simulink model "T2F_IEEE34bus_v2019b_Phasor_PI_ZIPload"  (R2024a)
settings: Solver=ode4  StartTime=0.0  StopTime=60  FixedStep=Ts  MaxStep=1e-4  RelTol=1e-4
InitFcn:
  | a=1; % Loading Factor
  | Ts=0.1;% For Delay Blocks in Voltage Regulator Controls
  | % phase to sequence conversion of RXB matrices
  | c=1*exp(sqrt(-1)*(120*pi/180));
  | T=[1 1 1;1 c*c c;1 c c*c];
  | Tinv=1/3*[1 1 1;1 c c*c;1 c*c c];
  | 
  | % Simulation data for the IEEE 34 Node Test Feeder model
  | mi2km = 1.60934;%  miles to km conversion
  | ft2km = 0.0003048; % feet to km conversion
  | ms2F = 1*1e-6/(2*pi*60);% microsiemens to Farads conversion
  | 
  | %% Configuration 300 - series reactance - ohm/mile
  | R_300 = [1.3368 0.2101 0.2130;0.2101 1.3238 0.2066;0.2130 0.2066 1.3294];
  | X_300 = [1.3343 0.5779 0.5015;0.5779 1.3569 0.4591;0.5015 0.4591 1.3471];
  | % charging susceptance - microsiemens/mile
  | B_300 = [5.3350 -1.5313 -0.9943;-1.5313 5.0979 -0.6212;-0.9943 -0.6212 4.8880];
  | 
  | R_300 = R_300/mi2km;
  | Rseq=Tinv*R_300*T;
  | R1_300=Rseq(2,2);R0_300=Rseq(1,1);
  | 
  | L_300 = (X_300/(2*pi*60))/mi2km;
  | Lseq=Tinv*L_300*T;
  | L1_300=Lseq(2,2);L0_300=Lseq(1,1);
  | 
  | C_300 =(B_300*ms2F)/mi2km;
  | Cseq=Tinv*C_300*T;
  | C1_300=Cseq(2,2);C0_300=Cseq(1,1);
  | 
  | %% Configuration 301 - series reactance - ohm/mile
  | R_301 = [1.9300 0.2327 0.2359;0.2327 1.9157 0.2288;0.2359 0.2288 1.9219];
  | X_301 = [1.4115 0.6442 0.5691;0.6442 1.4281 0.5238;0.5691 0.5238 1.4209];
  | % charging susceptance - microsiemens/mile
  | B_301 = [5.1207 -1.4364 -0.9402;-1.4364 4.9055 -0.5951;-0.9402 -0.5951 4.7154];
  | 
  | R_301 = R_301/mi2km;
  | Rseq=Tinv*R_301*T;
  | R1_301=Rseq(2,2);R0_301=Rseq(1,1);
  | 
  | L_301 = (X_301/(2*pi*60))/mi2km;
  | Lseq=Tinv*L_301*T;
  | L1_301=Lseq(2,2);L0_301=Lseq(1,1);
  | 
  | C_301 =(B_301*ms2F)/mi2km;
  | Cseq=Tinv*C_301*T;
  | C1_301=Cseq(2,2);C0_301=Cseq(1,1);
  | 
  | %% Configuration 302 - series reactance - ohm/mile
  | R_302 = [2.7995 0 0;0 0 0;0 0 0];
  | X_302 = [1.4855 0 0;0 0 0;0 0 0];
  | % charging susceptance - microsiemens/mile
  | B_302 = [4.2251 0 0;0 0 0;0 0 0];
  | 
  | R_302 = R_302/mi2km;
  | Rseq=Tinv*R_302*T;
  | R1_302=Rseq(2,2);R0_302=Rseq(1,1);
  | 
  | L_302 = (X_302/(2*pi*60))/mi2km;
  | Lseq=Tinv*L_302*T;
  | ... (+41 lines)
values from neighbouring files (symbols this model uses):
  ccc1 = Ccc*d    [CarregaDados1km.m]
  ccc2 = Ccc*d    [CarregaDados1km.m]
  ccc3 = Ccc*d    [CarregaDados1km.m]
  cct1 = Cct*d    [CarregaDados1km.m]
  cct2 = Cct*d    [CarregaDados1km.m]
  cct3 = Cct*d    [CarregaDados1km.m]
  cequa1 = 0    [CarregaDados1km.m]
  cequa2 = 0    [CarregaDados1km.m]
  cequa3 = 0    [CarregaDados1km.m]
  le1 = 1e-10    [CarregaDados1km.m]
  lm1 = (imag(Zm)/(2*pi*f))*d    [CarregaDados1km.m]
  lm2 = (imag(Zm)/(2*pi*f))*d    [CarregaDados1km.m]
  lm3 = (imag(Zm)/(2*pi*f))*d    [CarregaDados1km.m]
  lp1 = (imag(Zp)/(2*pi*f))*d    [CarregaDados1km.m]
  lp2 = (imag(Zp)/(2*pi*f))*d    [CarregaDados1km.m]
  lp3 = (imag(Zp)/(2*pi*f))*d    [CarregaDados1km.m]
  NRE1 = 1e-12    [CarregaDados1km.m]
  rm1 = real(Zm)*d    [CarregaDados1km.m]
  rm2 = real(Zm)*d    [CarregaDados1km.m]
  rm3 = real(Zm)*d    [CarregaDados1km.m]
  rp1 = real(Zp)*d    [CarregaDados1km.m]
  rp2 = real(Zp)*d    [CarregaDados1km.m]
  rp3 = real(Zp)*d    [CarregaDados1km.m]
  rtc0 = 10    [CarregaDados1km.m]
  rtc1 = 10    [CarregaDados1km.m]
  rtc2 = 10    [CarregaDados1km.m]
  rtc3 = 10    [CarregaDados1km.m]
undefined symbols (not defined in the file or in its folder): D11, Delta, find_system, j, le, m1, m2, m3
libraries: spsSeriesRLCBranchLib x192, spsVoltageMeasurementLib x96, spsControlledCurrentSourceLib x90, spsGroundLib x87, spsPowerPhasorLib x57, spsThreePhaseVIMeasurementLib x37, spsThreePhasePISectionLineLib x20, spsCurrentMeasurementLib x12, spsOnDelayLib x12, spsMutualInductanceLib x10, spsThreePhaseSeriesRLCLoadLib x6, spsControlledVoltageSourceLib x6
(part 5 of 8)

== system T2F_IEEE34bus_v2019b_Phasor_PI_ZIPload/Regulator 1 ==
  Mux : Mux  Inputs=3
  Single Phase SVR_A : Subsystem  LoadFcn=find_system(gcs,'FollowLinks', 'on', 'LookUnderMasks', 'all');  mask(Single-Phase OLTC){pNom=5e6/3, fNom=60, vNom=24.9e3/sqrt(3), ctRatio=100, ptRatio=120, DeltaU=0.00625, TapMinMax=[-16 16], InitialTap=12, TapSelectionTime=8, RegulatorOn=on, Regulator=[122/120  2/120  2], Comp=[2.7 1.6]}
      mask prompts: pNom "Nominal Power (VA)"; fNom "Nominal Frequency (Hz)"; vNom "Nominal Voltage (Vrms)"; ctRatio "Primary CT Rating (A)"; ptRatio "PT Ratio"; DeltaU "Voltage Step Per Tap (pu)"; TapMinMax "Minimum and Maximum Tap Positions"; InitialTap "Initial Tap Position"; TapSelectionTime "Tap Selection Time (s)"; RegulatorOn "Voltage Regulator"; Regulator "Voltage Regulator [ Vref(pu) DeadBand(pu)  Delay(s)]"; Comp "Compensator Settings [R (V) X(V)]"
      mask help:
      | Models a single-phase On Load Tap Changer (OLTC). The single-phase secondary of multi-tap winding is modeled with a Variable-Ratio Transformer block.
      |
      | The transformer voltage ratio U2/U1 (in pu) is given by:
      |                 U2/U1= 1+TapPosition*DeltaU
      | Tap position 0 corresponds to nominal voltage ratio.
      |
      | When Voltage regulator is 'on',  voltage regulator asks for a tap change if:
      |                  abs(Vm-Vref)>DeadBand/2  during a time  t > Delay.
      |
      | where 'Vm' is voltage measured at regulating point and Vref is reference voltage.
      | With line drop compensation, Vm=Vsec-Isec(R+jX)
      mask init:
      | RegulatorVref=Regulator(1);
      | RegulatorDeadBand=Regulator(2);
      | RegulatorDelay=Regulator(3);
      | Rc=Comp(1);
      | Xc=Comp(2);
      mask TypeOptions RegulatorOn: off | on
      mask Callback RegulatorOn:
      | tempMaskVis=get_param(gcb,'MaskVisibilities');
      | if strcmp(get_param(gcb,'RegulatorOn'),'on')
      | 	tempMaskVis{11}='on';
      | 	set_param(gcb,'MaskVisibilities',tempMaskVis);
      | else
      | 	tempMaskVis{11}='off';
      | 	set_param(gcb,'MaskVisibilities',tempMaskVis);
      | end
      | if strcmp(get_param(gcb,'RegulatorOn'),'on')
      | 	tempMaskVis{12}='on';
      | 	set_param(gcb,'MaskVisibilities',tempMaskVis);
      | else
      | 	tempMaskVis{12}='off';
      | 	set_param(gcb,'MaskVisibilities',tempMaskVis);
      | end
      mask DialogControl Container8 Prompt: Setup
      mask DialogControl Container13 Prompt: Regulator Parameters
      mask Display:
      | color('blue');
      | r=50;x=40;y=80;
      | th = 0:pi/100:2*pi;
      | f = r * exp(j*th) + x+j*y;
      | plot(real(f), imag(f));
      | color('red');
      | plot([-10 90],[30,130])
      | plot([75 90],[125,130])
      | plot([85 90],[115,130])
      | color('black')
      | port_label('Lconn',1,'S');port_label('Rconn',1,'L');
  Single Phase SVR_B : Subsystem  LoadFcn=find_system(gcs,'FollowLinks', 'on', 'LookUnderMasks', 'all');  mask(Single-Phase OLTC){pNom=5e6/3, fNom=60, vNom=24.9e3/sqrt(3), ctRatio=100, ptRatio=120, DeltaU=0.00625, TapMinMax=[-16 16], InitialTap=5, TapSelectionTime=8, RegulatorOn=on, Regulator=[122/120  2/120  2], Comp=[2.7 1.6]}
      mask prompts: pNom "Nominal Power (VA)"; fNom "Nominal Frequency (Hz)"; vNom "Nominal Voltage (Vrms)"; ctRatio "Primary CT Rating (A)"; ptRatio "PT Ratio"; DeltaU "Voltage Step Per Tap (pu)"; TapMinMax "Minimum and Maximum Tap Positions"; InitialTap "Initial Tap Position"; TapSelectionTime "Tap Selection Time (s)"; RegulatorOn "Voltage Regulator"; Regulator "Voltage Regulator [ Vref(pu) DeadBand(pu)  Delay(s)]"; Comp "Compensator Settings [R (V) X(V)]"
      mask help:
      | Models a single-phase On Load Tap Changer (OLTC). The single-phase secondary of multi-tap winding is modeled with a Variable-Ratio Transformer block.
      |
      | The transformer voltage ratio U2/U1 (in pu) is given by:
      |                 U2/U1= 1+TapPosition*DeltaU
      | Tap position 0 corresponds to nominal voltage ratio.
      |
      | When Voltage regulator is 'on',  voltage regulator asks for a tap change if:
      |                  abs(Vm-Vref)>DeadBand/2  during a time  t > Delay.
      |
      | where 'Vm' is voltage measured at regulating point and Vref is reference voltage.
      | With line drop compensation, Vm=Vsec-Isec(R+jX)
      mask init:
      | RegulatorVref=Regulator(1);
      | RegulatorDeadBand=Regulator(2);
      | RegulatorDelay=Regulator(3);
      | Rc=Comp(1);
      | Xc=Comp(2);
      mask TypeOptions RegulatorOn: off | on
      mask Callback RegulatorOn:
      | tempMaskVis=get_param(gcb,'MaskVisibilities');
      | if strcmp(get_param(gcb,'RegulatorOn'),'on')
      | 	tempMaskVis{11}='on';
      | 	set_param(gcb,'MaskVisibilities',tempMaskVis);
      | else
      | 	tempMaskVis{11}='off';
      | 	set_param(gcb,'MaskVisibilities',tempMaskVis);
      | end
      | if strcmp(get_param(gcb,'RegulatorOn'),'on')
      | 	tempMaskVis{12}='on';
      | 	set_param(gcb,'MaskVisibilities',tempMaskVis);
      | else
      | 	tempMaskVis{12}='off';
      | 	set_param(gcb,'MaskVisibilities',tempMaskVis);
      | end
      mask DialogControl Container8 Prompt: Setup
      mask DialogControl Container13 Prompt: Regulator Parameters
      mask Display:
      | color('blue');
      | r=50;x=40;y=80;
      | th = 0:pi/100:2*pi;
      | f = r * exp(j*th) + x+j*y;
      | plot(real(f), imag(f));
      | color('red');
      | plot([-10 90],[30,130])
      | plot([75 90],[125,130])
      | plot([85 90],[115,130])
      | color('black')
      | port_label('Lconn',1,'S');port_label('Rconn',1,'L');
  Single Phase SVR_C : Subsystem  LoadFcn=find_system(gcs,'FollowLinks', 'on', 'LookUnderMasks', 'all');  mask(Single-Phase OLTC){pNom=5e6/3, fNom=60, vNom=24.9e3/sqrt(3), ctRatio=100, ptRatio=120, DeltaU=0.00625, TapMinMax=[-16 16], InitialTap=5, TapSelectionTime=8, RegulatorOn=on, Regulator=[122/120  2/120  2], Comp=[2.7 1.6]}
      mask prompts: pNom "Nominal Power (VA)"; fNom "Nominal Frequency (Hz)"; vNom "Nominal Voltage (Vrms)"; ctRatio "Primary CT Rating (A)"; ptRatio "PT Ratio"; DeltaU "Voltage Step Per Tap (pu)"; TapMinMax "Minimum and Maximum Tap Positions"; InitialTap "Initial Tap Position"; TapSelectionTime "Tap Selection Time (s)"; RegulatorOn "Voltage Regulator"; Regulator "Voltage Regulator [ Vref(pu) DeadBand(pu)  Delay(s)]"; Comp "Compensator Settings [R (V) X(V)]"
      mask help:
      | Models a single-phase On Load Tap Changer (OLTC). The single-phase secondary of multi-tap winding is modeled with a Variable-Ratio Transformer block.
      |
      | The transformer voltage ratio U2/U1 (in pu) is given by:
      |                 U2/U1= 1+TapPosition*DeltaU
      | Tap position 0 corresponds to nominal voltage ratio.
      |
      | When Voltage regulator is 'on',  voltage regulator asks for a tap change if:
      |                  abs(Vm-Vref)>DeadBand/2  during a time  t > Delay.
      |
      | where 'Vm' is voltage measured at regulating point and Vref is reference voltage.
      | With line drop compensation, Vm=Vsec-Isec(R+jX)
      mask init:
      | RegulatorVref=Regulator(1);
      | RegulatorDeadBand=Regulator(2);
      | RegulatorDelay=Regulator(3);
      | Rc=Comp(1);
      | Xc=Comp(2);
      mask TypeOptions RegulatorOn: off | on
      mask Callback RegulatorOn:
      | tempMaskVis=get_param(gcb,'MaskVisibilities');
      | if strcmp(get_param(gcb,'RegulatorOn'),'on')
      | 	tempMaskVis{11}='on';
      | 	set_param(gcb,'MaskVisibilities',tempMaskVis);
      | else
      | 	tempMaskVis{11}='off';
      | 	set_param(gcb,'MaskVisibilities',tempMaskVis);
      | end
      | if strcmp(get_param(gcb,'RegulatorOn'),'on')
      | 	tempMaskVis{12}='on';
      | 	set_param(gcb,'MaskVisibilities',tempMaskVis);
      | else
      | 	tempMaskVis{12}='off';
      | 	set_param(gcb,'MaskVisibilities',tempMaskVis);
      | end
      mask DialogControl Container8 Prompt: Setup
      mask DialogControl Container13 Prompt: Regulator Parameters
      mask Display:
      | color('blue');
      | r=50;x=40;y=80;
      | th = 0:pi/100:2*pi;
      | f = r * exp(j*th) + x+j*y;
      | plot(real(f), imag(f));
      | color('red');
      | plot([-10 90],[30,130])
      | plot([75 90],[125,130])
      | plot([85 90],[115,130])
      | color('black')
      | port_label('Lconn',1,'S');port_label('Rconn',1,'L');
  A : PMIOPort  Side=Left
  a : PMIOPort  Port=2  Side=Right
  B : PMIOPort  Port=3  Side=Left
  b : PMIOPort  Port=4  Side=Right
  C : PMIOPort  Port=5  Side=Left
  c : PMIOPort  Port=6  Side=Right
  Tap : Outport
  wires:
  Mux/1 -> Tap/1
  Single Phase SVR_C/1(Tap) -> Mux/3
  Single Phase SVR_B/1(Tap) -> Mux/2
  Single Phase SVR_A/1(Tap) -> Mux/1
  connections:
  Single Phase SVR_C/RConn1 -- c/RConn1
  Single Phase SVR_C/LConn1 -- C/RConn1
  Single Phase SVR_B/RConn1 -- b/RConn1
  Single Phase SVR_B/LConn1 -- B/RConn1
  Single Phase SVR_A/LConn1 -- A/RConn1
  Single Phase SVR_A/RConn1 -- a/RConn1

== system T2F_IEEE34bus_v2019b_Phasor_PI_ZIPload/Regulator 2 ==
  Mux : Mux  Inputs=3
  Single Phase SVR_A : Subsystem  LoadFcn=find_system(gcs,'FollowLinks', 'on', 'LookUnderMasks', 'all');  mask(Single-Phase OLTC){pNom=5e6/3, fNom=60, vNom=24.9e3/sqrt(3), ctRatio=100, ptRatio=120, DeltaU=0.00625, TapMinMax=[-16 16], InitialTap=13, TapSelectionTime=13, RegulatorOn=on, Regulator=[124/120  2/120  2], Comp=[2.5 1.5]}
      mask prompts: pNom "Nominal Power (VA)"; fNom "Nominal Frequency (Hz)"; vNom "Nominal Voltage (Vrms)"; ctRatio "Primary CT Rating (A)"; ptRatio "PT Ratio"; DeltaU "Voltage Step Per Tap (pu)"; TapMinMax "Minimum and Maximum Tap Positions"; InitialTap "Initial Tap Position"; TapSelectionTime "Tap Selection Time (s)"; RegulatorOn "Voltage Regulator"; Regulator "Voltage Regulator [ Vref(pu) DeadBand(pu)  Delay(s)]"; Comp "Compensator Settings [R (V) X(V)]"
      mask help:
      | Models a single-phase On Load Tap Changer (OLTC). The single-phase secondary of multi-tap winding is modeled with a Variable-Ratio Transformer block.
      |
      | The transformer voltage ratio U2/U1 (in pu) is given by:
      |                 U2/U1= 1+TapPosition*DeltaU
      | Tap position 0 corresponds to nominal voltage ratio.
      |
      | When Voltage regulator is 'on',  voltage regulator asks for a tap change if:
      |                  abs(Vm-Vref)>DeadBand/2  during a time  t > Delay.
      |
      | where 'Vm' is voltage measured at regulating point and Vref is reference voltage.
      | With line drop compensation, Vm=Vsec-Isec(R+jX)
      mask init:
      | RegulatorVref=Regulator(1);
      | RegulatorDeadBand=Regulator(2);
      | RegulatorDelay=Regulator(3);
      | Rc=Comp(1);
      | Xc=Comp(2);
      mask TypeOptions RegulatorOn: off | on
      mask Callback RegulatorOn:
      | tempMaskVis=get_param(gcb,'MaskVisibilities');
      | if strcmp(get_param(gcb,'RegulatorOn'),'on')
      | 	tempMaskVis{11}='on';
      | 	set_param(gcb,'MaskVisibilities',tempMaskVis);
      | else
      | 	tempMaskVis{11}='off';
      | 	set_param(gcb,'MaskVisibilities',tempMaskVis);
      | end
      | if strcmp(get_param(gcb,'RegulatorOn'),'on')
      | 	tempMaskVis{12}='on';
      | 	set_param(gcb,'MaskVisibilities',tempMaskVis);
      | else
      | 	tempMaskVis{12}='off';
      | 	set_param(gcb,'MaskVisibilities',tempMaskVis);
      | end
      mask DialogControl Container8 Prompt: Setup
      mask DialogControl Container13 Prompt: Regulator Parameters
      mask Display:
      | color('blue');
      | r=50;x=40;y=80;
      | th = 0:pi/100:2*pi;
      | f = r * exp(j*th) + x+j*y;
      | plot(real(f), imag(f));
      | color('red');
      | plot([-10 90],[30,130])
      | plot([75 90],[125,130])
      | plot([85 90],[115,130])
      | color('black')
      | port_label('Lconn',1,'S');port_label('Rconn',1,'L');
  Single Phase SVR_B : Subsystem  LoadFcn=find_system(gcs,'FollowLinks', 'on', 'LookUnderMasks', 'all');  mask(Single-Phase OLTC){pNom=5e6/3, fNom=60, vNom=24.9e3/sqrt(3), ctRatio=100, ptRatio=120, DeltaU=0.00625, TapMinMax=[-16 16], InitialTap=11, TapSelectionTime=13, RegulatorOn=on, Regulator=[124/120  2/120  2], Comp=[2.5 1.5]}
      mask prompts: pNom "Nominal Power (VA)"; fNom "Nominal Frequency (Hz)"; vNom "Nominal Voltage (Vrms)"; ctRatio "Primary CT Rating (A)"; ptRatio "PT Ratio"; DeltaU "Voltage Step Per Tap (pu)"; TapMinMax "Minimum and Maximum Tap Positions"; InitialTap "Initial Tap Position"; TapSelectionTime "Tap Selection Time (s)"; RegulatorOn "Voltage Regulator"; Regulator "Voltage Regulator [ Vref(pu) DeadBand(pu)  Delay(s)]"; Comp "Compensator Settings [R (V) X(V)]"
      mask help:
      | Models a single-phase On Load Tap Changer (OLTC). The single-phase secondary of multi-tap winding is modeled with a Variable-Ratio Transformer block.
      |
      | The transformer voltage ratio U2/U1 (in pu) is given by:
      |                 U2/U1= 1+TapPosition*DeltaU
      | Tap position 0 corresponds to nominal voltage ratio.
      |
      | When Voltage regulator is 'on',  voltage regulator asks for a tap change if:
      |                  abs(Vm-Vref)>DeadBand/2  during a time  t > Delay.
      |
      | where 'Vm' is voltage measured at regulating point and Vref is reference voltage.
      | With line drop compensation, Vm=Vsec-Isec(R+jX)
      mask init:
      | RegulatorVref=Regulator(1);
      | RegulatorDeadBand=Regulator(2);
      | RegulatorDelay=Regulator(3);
      | Rc=Comp(1);
      | Xc=Comp(2);
      mask TypeOptions RegulatorOn: off | on
      mask Callback RegulatorOn:
      | tempMaskVis=get_param(gcb,'MaskVisibilities');
      | if strcmp(get_param(gcb,'RegulatorOn'),'on')
      | 	tempMaskVis{11}='on';
      | 	set_param(gcb,'MaskVisibilities',tempMaskVis);
      | else
      | 	tempMaskVis{11}='off';
      | 	set_param(gcb,'MaskVisibilities',tempMaskVis);
      | end
      | if strcmp(get_param(gcb,'RegulatorOn'),'on')
      | 	tempMaskVis{12}='on';
      | 	set_param(gcb,'MaskVisibilities',tempMaskVis);
      | else
      | 	tempMaskVis{12}='off';
      | 	set_param(gcb,'MaskVisibilities',tempMaskVis);
      | end
      mask DialogControl Container8 Prompt: Setup
      mask DialogControl Container13 Prompt: Regulator Parameters
      mask Display:
      | color('blue');
      | r=50;x=40;y=80;
      | th = 0:pi/100:2*pi;
      | f = r * exp(j*th) + x+j*y;
      | plot(real(f), imag(f));
      | color('red');
      | plot([-10 90],[30,130])
      | plot([75 90],[125,130])
      | plot([85 90],[115,130])
      | color('black')
      | port_label('Lconn',1,'S');port_label('Rconn',1,'L');
  Single Phase SVR_C : Subsystem  LoadFcn=find_system(gcs,'FollowLinks', 'on', 'LookUnderMasks', 'all');  mask(Single-Phase OLTC){pNom=5e6/3, fNom=60, vNom=24.9e3/sqrt(3), ctRatio=100, ptRatio=120, DeltaU=0.00625, TapMinMax=[-16 16], InitialTap=12, TapSelectionTime=13, RegulatorOn=on, Regulator=[124/120  2/120  2], Comp=[2.5 1.5]}
      mask prompts: pNom "Nominal Power (VA)"; fNom "Nominal Frequency (Hz)"; vNom "Nominal Voltage (Vrms)"; ctRatio "Primary CT Rating (A)"; ptRatio "PT Ratio"; DeltaU "Voltage Step Per Tap (pu)"; TapMinMax "Minimum and Maximum Tap Positions"; InitialTap "Initial Tap Position"; TapSelectionTime "Tap Selection Time (s)"; RegulatorOn "Voltage Regulator"; Regulator "Voltage Regulator [ Vref(pu) DeadBand(pu)  Delay(s)]"; Comp "Compensator Settings [R (V) X(V)]"
      mask help:
      | Models a single-phase On Load Tap Changer (OLTC). The single-phase secondary of multi-tap winding is modeled with a Variable-Ratio Transformer block.
      |
      | The transformer voltage ratio U2/U1 (in pu) is given by:
      |                 U2/U1= 1+TapPosition*DeltaU
      | Tap position 0 corresponds to nominal voltage ratio.
      |
      | When Voltage regulator is 'on',  voltage regulator asks for a tap change if:
      |                  abs(Vm-Vref)>DeadBand/2  during a time  t > Delay.
      |
      | where 'Vm' is voltage measured at regulating point and Vref is reference voltage.
      | With line drop compensation, Vm=Vsec-Isec(R+jX)
      mask init:
      | RegulatorVref=Regulator(1);
      | RegulatorDeadBand=Regulator(2);
      | RegulatorDelay=Regulator(3);
      | Rc=Comp(1);
      | Xc=Comp(2);
      mask TypeOptions RegulatorOn: off | on
      mask Callback RegulatorOn:
      | tempMaskVis=get_param(gcb,'MaskVisibilities');
      | if strcmp(get_param(gcb,'RegulatorOn'),'on')
      | 	tempMaskVis{11}='on';
      | 	set_param(gcb,'MaskVisibilities',tempMaskVis);
      | else
      | 	tempMaskVis{11}='off';
      | 	set_param(gcb,'MaskVisibilities',tempMaskVis);
      | end
      | if strcmp(get_param(gcb,'RegulatorOn'),'on')
      | 	tempMaskVis{12}='on';
      | 	set_param(gcb,'MaskVisibilities',tempMaskVis);
      | else
      | 	tempMaskVis{12}='off';
      | 	set_param(gcb,'MaskVisibilities',tempMaskVis);
      | end
      mask DialogControl Container8 Prompt: Setup
      mask DialogControl Container13 Prompt: Regulator Parameters
      mask Display:
      | color('blue');
      | r=50;x=40;y=80;
      | th = 0:pi/100:2*pi;
      | f = r * exp(j*th) + x+j*y;
      | plot(real(f), imag(f));
      | color('red');
      | plot([-10 90],[30,130])
      | plot([75 90],[125,130])
      | plot([85 90],[115,130])
      | color('black')
      | port_label('Lconn',1,'S');port_label('Rconn',1,'L');
  A : PMIOPort  Side=Left
  a : PMIOPort  Port=2  Side=Right
  B : PMIOPort  Port=3  Side=Left
  b : PMIOPort  Port=4  Side=Right
  C : PMIOPort  Port=5  Side=Left
  c : PMIOPort  Port=6  Side=Right
  Tap : Outport
  wires:
  Mux/1 -> Tap/1
  Single Phase SVR_C/1(Tap) -> Mux/3
  Single Phase SVR_B/1(Tap) -> Mux/2
  Single Phase SVR_A/1(Tap) -> Mux/1
  connections:
  Single Phase SVR_C/RConn1 -- c/RConn1
  Single Phase SVR_C/LConn1 -- C/RConn1
  Single Phase SVR_B/RConn1 -- b/RConn1
  Single Phase SVR_B/LConn1 -- B/RConn1
  Single Phase SVR_A/LConn1 -- A/RConn1
  Single Phase SVR_A/RConn1 -- a/RConn1

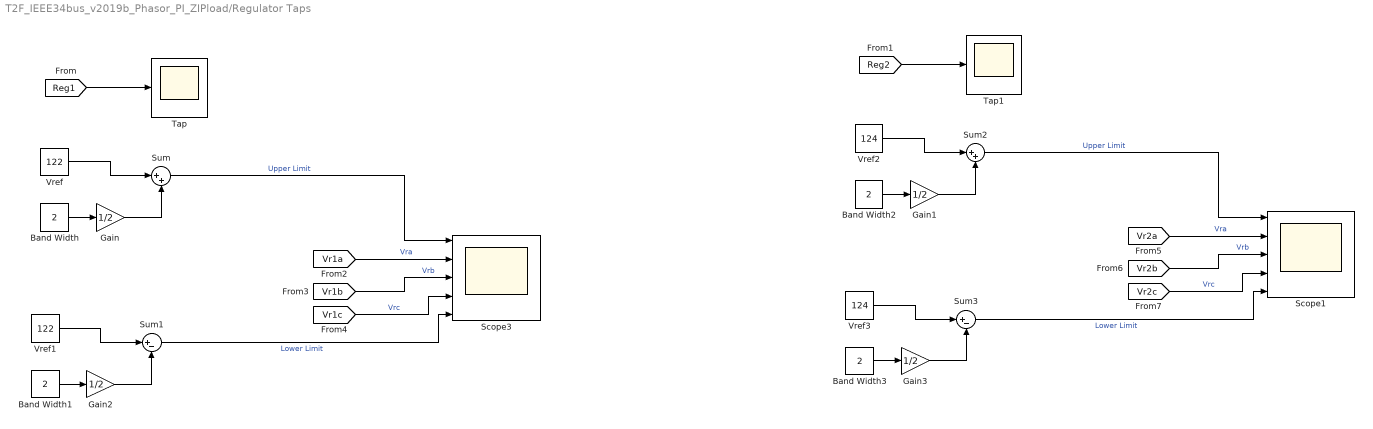
== system T2F_IEEE34bus_v2019b_Phasor_PI_ZIPload/Regulator Taps ==
  Band Width{,1..3} (4 alike) : Constant  Value=2
  Gain{,1..3} (4 alike) : Gain  Gain=1/2
  Scope1 : Scope  NumInputPorts=5
  Scope3 : Scope  NumInputPorts=5
  Sum : Sum  Inputs=|++
  Sum1 : Sum  Inputs=|+-
  Sum2 : Sum  Inputs=|++
  Sum3 : Sum  Inputs=|+-
  Tap : Scope
  Tap1 : Scope
  Vref : Constant  Value=122
  Vref1 : Constant  Value=122
  Vref2 : Constant  Value=124
  Vref3 : Constant  Value=124
  wires:
  Vref/1 -> Sum/1
  Gain2/1 -> Sum1/2
  Band Width/1 -> Gain/1
  Gain/1 -> Sum/2
  [Reg1] -> Tap/1
  [Vr1c] -> Scope3/4  "Vrc"
  Band Width1/1 -> Gain2/1
  Sum/1 -> Scope3/1  "Upper Limit"
  Vref1/1 -> Sum1/1
  Sum1/1 -> Scope3/5  "Lower Limit"
  [Vr1b] -> Scope3/3  "Vrb"
  [Vr1a] -> Scope3/2  "Vra"
  [Vr2a] -> Scope1/2  "Vra"
  [Vr2b] -> Scope1/3  "Vrb"
  Sum3/1 -> Scope1/5  "Lower Limit"
  Vref3/1 -> Sum3/1
  Sum2/1 -> Scope1/1  "Upper Limit"
  Band Width3/1 -> Gain3/1
  [Vr2c] -> Scope1/4  "Vrc"
  [Reg2] -> Tap1/1
  Gain1/1 -> Sum2/2
  Band Width2/1 -> Gain1/1
  Gain3/1 -> Sum3/2
  Vref2/1 -> Sum2/1

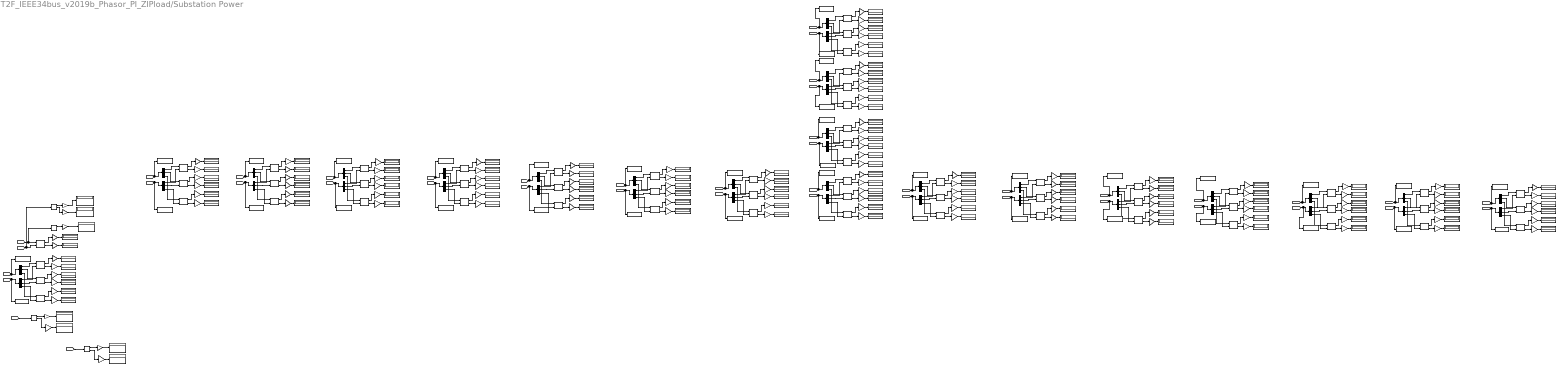
== system T2F_IEEE34bus_v2019b_Phasor_PI_ZIPload/Substation Power ==
  note: SYSTEM PHASE PHASE PHASE TOTAL
      | INPUT -------(A)-------|-------(B)-------|-------(C)-------|-------------------
      | kW : 759.136 | 666.663 | 617.072 | 2042.872
      | kVAr : 171.727 | 90.137 | 28.394 | 290.258
  note: PHASE C
  note: PHASE A
  note: PHASE B
  note: TOTAL
  note: Current 800- 802 AMP/DG
      | -------(A)-------|---------(B)----------|-------(C)-------
      | 51.56 -12.74 44.57 -127.70 40.92 117.37
  note: PHASE A
  note: PHASE B
  note: PHASE C
  note: PHASE B
  note: PHASE A
  note: PHASE C
  note: PHASE C
  note: PHASE B
  note: PHASE A
  note: PHASE A
  note: PHASE B
  note: PHASE C
  note: PHASE B
  note: PHASE A
  note: PHASE C
  note: PHASE C
  note: PHASE A
  note: PHASE B
  note: PHASE A
  note: PHASE B
  note: PHASE C
  note: PHASE B
  note: PHASE A
  note: PHASE C
  note: PHASE A
  note: PHASE C
  note: PHASE B
  note: PHASE C
  note: PHASE A
  note: PHASE B
  note: PHASE C
  note: PHASE B
  note: PHASE A
  note: PHASE B
  note: PHASE A
  note: PHASE C
  note: PHASE A
  note: PHASE B
  note: PHASE C
  note: PHASE A
  note: PHASE B
  note: PHASE C
  note: PHASE A
  note: PHASE C
  note: PHASE B
  note: PHASE A
  note: PHASE C
  note: PHASE B
  note: PHASE B
  note: PHASE C
  note: PHASE A
  note: PHASE B
  note: PHASE C
  note: PHASE A
  Complex to Magnitude-Angle{,1..3} (4 alike) : ComplexToMagnitudeAngle
  Demux{,1..37} (38 alike) : Demux  Outputs=3
  Display{,1..98,100..122,137} (123 alike) : Display
  Gain{,1..7,15..98,100..122,137} (116 alike) : Gain  Gain=1e-3
  Gain10 : Gain  Gain=180/pi
  Gain11 : Gain  Gain=1/sqrt(2)
  Gain12 : Gain  Gain=180/pi
  Gain13 : Gain  Gain=1/sqrt(2)
  Gain14 : Gain  Gain=180/pi
  Gain8 : Gain  Gain=1/(24900/sqrt(3))*1/sqrt(2)
  Gain9 : Gain  Gain=1/sqrt(2)
  "Power (3ph, Phasor)" : spsPower3phPhasorLib/Power (3ph, Phasor)
      settings: LibrarySourceBlock=|
      | sps_lib/Sensors and Measurements/Power
      | (3ph, Phasor)
  Power (Phasor){,1..56} (57 alike) : spsPowerPhasorLib/Power (Phasor)
      settings: LibrarySourceBlock=|
      | sps_lib/Sensors and Measurements/Power
      | (Phasor)
  To Workspace : ToWorkspace  VariableName=V802  SampleTime=-1
      settings: MaxDataPoints=1  Save2DSignal=2-D array (concatenate along first dimension)
  To Workspace1 : ToWorkspace  VariableName=I802  SampleTime=-1
      settings: MaxDataPoints=1  Save2DSignal=2-D array (concatenate along first dimension)
  To Workspace10 : ToWorkspace  VariableName=VRG10  SampleTime=-1
      settings: MaxDataPoints=1  Save2DSignal=2-D array (concatenate along first dimension)
  To Workspace11 : ToWorkspace  VariableName=IRG10  SampleTime=-1
      settings: MaxDataPoints=1  Save2DSignal=2-D array (concatenate along first dimension)
  To Workspace12 : ToWorkspace  VariableName=V850  SampleTime=-1
      settings: MaxDataPoints=1  Save2DSignal=2-D array (concatenate along first dimension)
  To Workspace13 : ToWorkspace  VariableName=I850  SampleTime=-1
      settings: MaxDataPoints=1  Save2DSignal=2-D array (concatenate along first dimension)
  To Workspace14 : ToWorkspace  VariableName=V816  SampleTime=-1
      settings: MaxDataPoints=1  Save2DSignal=2-D array (concatenate along first dimension)
  To Workspace15 : ToWorkspace  VariableName=I816  SampleTime=-1
      settings: MaxDataPoints=1  Save2DSignal=2-D array (concatenate along first dimension)
  To Workspace16 : ToWorkspace  VariableName=V818  SampleTime=-1
      settings: MaxDataPoints=1  Save2DSignal=2-D array (concatenate along first dimension)
  To Workspace17 : ToWorkspace  VariableName=I818  SampleTime=-1
      settings: MaxDataPoints=1  Save2DSignal=2-D array (concatenate along first dimension)
  To Workspace18 : ToWorkspace  VariableName=V820  SampleTime=-1
      settings: MaxDataPoints=1  Save2DSignal=2-D array (concatenate along first dimension)
  To Workspace19 : ToWorkspace  VariableName=I820  SampleTime=-1
      settings: MaxDataPoints=1  Save2DSignal=2-D array (concatenate along first dimension)
  To Workspace2 : ToWorkspace  VariableName=V806  SampleTime=-1
      settings: MaxDataPoints=1  Save2DSignal=2-D array (concatenate along first dimension)
  To Workspace20 : ToWorkspace  VariableName=V822  SampleTime=-1
      settings: MaxDataPoints=1  Save2DSignal=2-D array (concatenate along first dimension)
  To Workspace21 : ToWorkspace  VariableName=I822  SampleTime=-1
      settings: MaxDataPoints=1  Save2DSignal=2-D array (concatenate along first dimension)
  To Workspace22 : ToWorkspace  VariableName=V824  SampleTime=-1
      settings: MaxDataPoints=1  Save2DSignal=2-D array (concatenate along first dimension)
  To Workspace23 : ToWorkspace  VariableName=I824  SampleTime=-1
      settings: MaxDataPoints=1  Save2DSignal=2-D array (concatenate along first dimension)
  To Workspace24 : ToWorkspace  VariableName=V828  SampleTime=-1
      settings: MaxDataPoints=1  Save2DSignal=2-D array (concatenate along first dimension)
  To Workspace25 : ToWorkspace  VariableName=I828  SampleTime=-1
      settings: MaxDataPoints=1  Save2DSignal=2-D array (concatenate along first dimension)
  To Workspace26 : ToWorkspace  VariableName=V830  SampleTime=-1
      settings: MaxDataPoints=1  Save2DSignal=2-D array (concatenate along first dimension)
  To Workspace27 : ToWorkspace  VariableName=I830  SampleTime=-1
      settings: MaxDataPoints=1  Save2DSignal=2-D array (concatenate along first dimension)
  To Workspace28 : ToWorkspace  VariableName=V854  SampleTime=-1
      settings: MaxDataPoints=1  Save2DSignal=2-D array (concatenate along first dimension)
  To Workspace29 : ToWorkspace  VariableName=I854  SampleTime=-1
      settings: MaxDataPoints=1  Save2DSignal=2-D array (concatenate along first dimension)
  To Workspace3 : ToWorkspace  VariableName=I806  SampleTime=-1
      settings: MaxDataPoints=1  Save2DSignal=2-D array (concatenate along first dimension)
  To Workspace30 : ToWorkspace  VariableName=V852  SampleTime=-1
      settings: MaxDataPoints=1  Save2DSignal=2-D array (concatenate along first dimension)
  To Workspace31 : ToWorkspace  VariableName=I852  SampleTime=-1
      settings: MaxDataPoints=1  Save2DSignal=2-D array (concatenate along first dimension)
  To Workspace32 : ToWorkspace  VariableName=VRG11  SampleTime=-1
      settings: MaxDataPoints=1  Save2DSignal=2-D array (concatenate along first dimension)
  To Workspace33 : ToWorkspace  VariableName=IRG11  SampleTime=-1
      settings: MaxDataPoints=1  Save2DSignal=2-D array (concatenate along first dimension)
  To Workspace34 : ToWorkspace  VariableName=V832  SampleTime=-1
      settings: MaxDataPoints=1  Save2DSignal=2-D array (concatenate along first dimension)
  To Workspace35 : ToWorkspace  VariableName=I832  SampleTime=-1
      settings: MaxDataPoints=1  Save2DSignal=2-D array (concatenate along first dimension)
  To Workspace36 : ToWorkspace  VariableName=V800  SampleTime=-1
      settings: MaxDataPoints=1  Save2DSignal=2-D array (concatenate along first dimension)
  To Workspace37 : ToWorkspace  VariableName=I800  SampleTime=-1
      settings: MaxDataPoints=1  Save2DSignal=2-D array (concatenate along first dimension)
  To Workspace4 : ToWorkspace  VariableName=V808  SampleTime=-1
      settings: MaxDataPoints=1  Save2DSignal=2-D array (concatenate along first dimension)
  To Workspace5 : ToWorkspace  VariableName=I808  SampleTime=-1
      settings: MaxDataPoints=1  Save2DSignal=2-D array (concatenate along first dimension)
  To Workspace6 : ToWorkspace  VariableName=V812  SampleTime=-1
      settings: MaxDataPoints=1  Save2DSignal=2-D array (concatenate along first dimension)
  To Workspace7 : ToWorkspace  VariableName=I812  SampleTime=-1
      settings: MaxDataPoints=1  Save2DSignal=2-D array (concatenate along first dimension)
  To Workspace8 : ToWorkspace  VariableName=V814  SampleTime=-1
      settings: MaxDataPoints=1  Save2DSignal=2-D array (concatenate along first dimension)
  To Workspace9 : ToWorkspace  VariableName=I814  SampleTime=-1
      settings: MaxDataPoints=1  Save2DSignal=2-D array (concatenate along first dimension)
  wires:
  "Power (3ph, Phasor)"/1 -> Gain/1
  "Power (3ph, Phasor)"/2 -> Gain1/1
  [V800] -> To Workspace36/1, Demux/1
  [I800] -> To Workspace37/1, Demux1/1
  Demux/1 -> Power (Phasor)/1
  Demux1/1 -> Power (Phasor)/2
  Demux/2 -> Power (Phasor)1/1
  Demux1/2 -> Power (Phasor)1/2
  Demux/3 -> Power (Phasor)2/1
  Demux1/3 -> Power (Phasor)2/2
  Power (Phasor)/1 -> Gain2/1
  Power (Phasor)/2 -> Gain3/1
  Power (Phasor)1/1 -> Gain4/1
  Power (Phasor)1/2 -> Gain5/1
  Power (Phasor)2/1 -> Gain6/1
  Power (Phasor)2/2 -> Gain7/1
  Gain/1 -> Display/1
  Gain1/1 -> Display1/1
  Gain2/1 -> Display2/1
  Gain3/1 -> Display3/1
  Gain4/1 -> Display4/1
  Gain5/1 -> Display5/1
  Gain6/1 -> Display6/1
  Gain7/1 -> Display7/1
  Complex to Magnitude-Angle/1 -> Gain8/1
  [V800] -> Complex to Magnitude-Angle/1, "Power (3ph, Phasor)"/1
  Gain8/1 -> Display8/1
  Gain9/1 -> Display9/1
  [I800] -> Complex to Magnitude-Angle1/1, "Power (3ph, Phasor)"/2
  Complex to Magnitude-Angle1/1 -> Gain9/1
  Complex to Magnitude-Angle1/2 -> Gain10/1
  Gain10/1 -> Display10/1
  Complex to Magnitude-Angle2/1 -> Gain11/1
  Gain12/1 -> Display11/1
  Complex to Magnitude-Angle2/2 -> Gain12/1
  [I800] -> Complex to Magnitude-Angle2/1
  Gain11/1 -> Display12/1
  Gain13/1 -> Display14/1
  Complex to Magnitude-Angle3/1 -> Gain13/1
  Gain14/1 -> Display13/1
  Complex to Magnitude-Angle3/2 -> Gain14/1
  [V818] -> Complex to Magnitude-Angle3/1
  Power (Phasor)4/2 -> Gain18/1
  Gain15/1 -> Display15/1
  Power (Phasor)3/2 -> Gain16/1
  Gain18/1 -> Display18/1
  Power (Phasor)4/1 -> Gain17/1
  Demux3/3 -> Power (Phasor)5/2
  Gain16/1 -> Display16/1
  Demux3/1 -> Power (Phasor)3/2
  Power (Phasor)5/2 -> Gain20/1
  Power (Phasor)5/1 -> Gain19/1
  Demux2/1 -> Power (Phasor)3/1
  Gain19/1 -> Display19/1
  Gain17/1 -> Display17/1
  Power (Phasor)3/1 -> Gain15/1
  Gain20/1 -> Display20/1
  Demux3/2 -> Power (Phasor)4/2
  Demux2/3 -> Power (Phasor)5/1
  Demux2/2 -> Power (Phasor)4/1
  [I802] -> To Workspace1/1, Demux3/1
  [V802] -> To Workspace/1, Demux2/1
  Demux4/3 -> Power (Phasor)8/1
  Demux4/2 -> Power (Phasor)7/1
  [I806] -> To Workspace3/1, Demux5/1
  Demux5/2 -> Power (Phasor)7/2
  [V806] -> To Workspace2/1, Demux4/1
  Gain24/1 -> Display24/1
  Power (Phasor)6/2 -> Gain22/1
  Gain23/1 -> Display23/1
  Gain25/1 -> Display25/1
  Power (Phasor)7/1 -> Gain23/1
  Gain22/1 -> Display22/1
  Demux5/3 -> Power (Phasor)8/2
  Demux4/1 -> Power (Phasor)6/1
  Demux5/1 -> Power (Phasor)6/2
  Gain26/1 -> Display26/1
  Power (Phasor)8/2 -> Gain26/1
  Power (Phasor)6/1 -> Gain21/1
  Gain21/1 -> Display21/1
  Power (Phasor)7/2 -> Gain24/1
  Power (Phasor)8/1 -> Gain25/1
  Power (Phasor)11/1 -> Gain31/1
  Gain27/1 -> Display27/1
  Gain28/1 -> Display28/1
  Power (Phasor)9/1 -> Gain27/1
  Power (Phasor)10/2 -> Gain30/1
  Gain32/1 -> Display32/1
  Demux6/1 -> Power (Phasor)9/1
  Demux7/1 -> Power (Phasor)9/2
  Demux7/3 -> Power (Phasor)11/2
  Power (Phasor)11/2 -> Gain32/1
  Gain31/1 -> Display31/1
  Gain29/1 -> Display29/1
  Power (Phasor)9/2 -> Gain28/1
  [V808] -> To Workspace4/1, Demux6/1
  Gain30/1 -> Display30/1
  [I808] -> To Workspace5/1, Demux7/1
  Power (Phasor)10/1 -> Gain29/1
  Demux6/3 -> Power (Phasor)11/1
  Demux7/2 -> Power (Phasor)10/2
  Demux6/2 -> Power (Phasor)10/1
  Demux8/3 -> Power (Phasor)13/1
  Power (Phasor)12/1 -> Gain35/1
  Demux9/2 -> Power (Phasor)12/2
  [I812] -> To Workspace7/1, Demux9/1
  Gain37/1 -> Display37/1
  Power (Phasor)13/2 -> Gain38/1
  Demux9/1 -> Power (Phasor)14/2
  Demux9/3 -> Power (Phasor)13/2
  Demux8/2 -> Power (Phasor)12/1
  Gain38/1 -> Display38/1
  Gain36/1 -> Display36/1
  Power (Phasor)14/2 -> Gain34/1
  Gain35/1 -> Display35/1
  Power (Phasor)12/2 -> Gain36/1
  Demux8/1 -> Power (Phasor)14/1
  [V812] -> To Workspace6/1, Demux8/1
  Gain33/1 -> Display33/1
  Power (Phasor)13/1 -> Gain37/1
  Power (Phasor)14/1 -> Gain33/1
  Gain34/1 -> Display34/1
  [V814] -> To Workspace8/1, Demux10/1
  Gain39/1 -> Display39/1
  Power (Phasor)16/1 -> Gain43/1
  Power (Phasor)17/1 -> Gain39/1
  Power (Phasor)15/2 -> Gain42/1
  Demux10/2 -> Power (Phasor)15/1
  Demux11/2 -> Power (Phasor)15/2
  Gain43/1 -> Display43/1
  Gain41/1 -> Display41/1
  Power (Phasor)17/2 -> Gain40/1
  Demux11/1 -> Power (Phasor)17/2
  [I814] -> To Workspace9/1, Demux11/1
  Power (Phasor)16/2 -> Gain44/1
  Gain44/1 -> Display44/1
  Demux10/3 -> Power (Phasor)16/1
  Demux10/1 -> Power (Phasor)17/1
  Power (Phasor)15/1 -> Gain41/1
  Demux11/3 -> Power (Phasor)16/2
  Gain42/1 -> Display42/1
  Gain40/1 -> Display40/1
  Gain45/1 -> Display45/1
  [VRG10] -> To Workspace10/1, Demux12/1
  Demux12/3 -> Power (Phasor)19/1
  Demux13/1 -> Power (Phasor)20/2
  Gain50/1 -> Display50/1
  Power (Phasor)19/2 -> Gain50/1
  [IRG10] -> To Workspace11/1, Demux13/1
  Gain46/1 -> Display46/1
  Gain48/1 -> Display48/1
  Demux13/3 -> Power (Phasor)19/2
  Gain49/1 -> Display49/1
  Power (Phasor)18/1 -> Gain47/1
  Demux13/2 -> Power (Phasor)18/2
  Power (Phasor)19/1 -> Gain49/1
  Demux12/1 -> Power (Phasor)20/1
  Power (Phasor)18/2 -> Gain48/1
  Gain47/1 -> Display47/1
  Power (Phasor)20/1 -> Gain45/1
  Demux12/2 -> Power (Phasor)18/1
  Power (Phasor)20/2 -> Gain46/1
  Gain53/1 -> Display53/1
  Power (Phasor)21/1 -> Gain53/1
  Demux14/2 -> Power (Phasor)21/1
  Gain54/1 -> Display54/1
  Power (Phasor)23/1 -> Gain51/1
  Power (Phasor)21/2 -> Gain54/1
  Demux15/2 -> Power (Phasor)21/2
  Gain52/1 -> Display52/1
  Demux15/3 -> Power (Phasor)22/2
  Power (Phasor)22/1 -> Gain55/1
  Demux15/1 -> Power (Phasor)23/2
  Gain56/1 -> Display56/1
  Power (Phasor)22/2 -> Gain56/1
  Power (Phasor)23/2 -> Gain52/1
  Gain55/1 -> Display55/1
  Demux14/3 -> Power (Phasor)22/1
  [V850] -> To Workspace12/1, Demux14/1
  Gain51/1 -> Display51/1
  [I850] -> To Workspace13/1, Demux15/1
  Demux14/1 -> Power (Phasor)23/1
  Demux17/1 -> Power (Phasor)26/2
  Power (Phasor)25/1 -> Gain61/1
  Demux17/3 -> Power (Phasor)25/2
  Demux16/2 -> Power (Phasor)24/1
  Power (Phasor)24/1 -> Gain59/1
  Gain60/1 -> Display60/1
  Demux17/2 -> Power (Phasor)24/2
  Power (Phasor)24/2 -> Gain60/1
  Gain59/1 -> Display59/1
  Demux16/3 -> Power (Phasor)25/1
  Power (Phasor)26/2 -> Gain58/1
  Gain57/1 -> Display57/1
  Gain58/1 -> Display58/1
  Gain62/1 -> Display62/1
  [V816] -> To Workspace14/1, Demux16/1
  Power (Phasor)25/2 -> Gain62/1
  Power (Phasor)26/1 -> Gain57/1
  Demux16/1 -> Power (Phasor)26/1
  [I816] -> To Workspace15/1, Demux17/1
  Gain61/1 -> Display61/1
  Demux18/1 -> Power (Phasor)29/1
  Gain63/1 -> Display63/1
  Power (Phasor)29/2 -> Gain64/1
  [I824] -> To Workspace23/1, Demux19/1
  Power (Phasor)29/1 -> Gain63/1
  Gain64/1 -> Display64/1
  Power (Phasor)28/2 -> Gain68/1
  Gain68/1 -> Display68/1
  [V824] -> To Workspace22/1, Demux18/1
  Gain67/1 -> Display67/1
  Gain65/1 -> Display65/1
  Demux19/2 -> Power (Phasor)27/2
  Demux18/2 -> Power (Phasor)27/1
  Demux18/3 -> Power (Phasor)28/1
  Power (Phasor)27/2 -> Gain66/1
  Demux19/1 -> Power (Phasor)29/2
  Power (Phasor)28/1 -> Gain67/1
  Demux19/3 -> Power (Phasor)28/2
  Power (Phasor)27/1 -> Gain65/1
  Gain66/1 -> Display66/1
  Demux20/2 -> Power (Phasor)30/1
  Gain71/1 -> Display71/1
  Demux21/3 -> Power (Phasor)31/2
  Demux21/2 -> Power (Phasor)30/2
  Demux20/3 -> Power (Phasor)31/1
  Gain72/1 -> Display72/1
  Demux21/1 -> Power (Phasor)32/2
  Power (Phasor)30/2 -> Gain72/1
  Power (Phasor)30/1 -> Gain71/1
  Gain70/1 -> Display70/1
  Power (Phasor)31/1 -> Gain73/1
  [I828] -> To Workspace25/1, Demux21/1
  Power (Phasor)32/1 -> Gain69/1
  Gain73/1 -> Display73/1
  Demux20/1 -> Power (Phasor)32/1
  Power (Phasor)31/2 -> Gain74/1
  [V828] -> To Workspace24/1, Demux20/1
  Gain74/1 -> Display74/1
  Gain69/1 -> Display69/1
  Power (Phasor)32/2 -> Gain70/1
  Gain76/1 -> Display76/1
  Power (Phasor)33/1 -> Gain77/1
  Power (Phasor)33/2 -> Gain78/1
  Demux23/1 -> Power (Phasor)35/2
  Gain78/1 -> Display78/1
  Demux22/3 -> Power (Phasor)34/1
  Gain77/1 -> Display77/1
  Demux23/3 -> Power (Phasor)34/2
  Demux23/2 -> Power (Phasor)33/2
  Gain80/1 -> Display80/1
  [V830] -> To Workspace26/1, Demux22/1
  Gain79/1 -> Display79/1
  Demux22/2 -> Power (Phasor)33/1
  Gain75/1 -> Display75/1
  Power (Phasor)35/1 -> Gain75/1
  Power (Phasor)34/2 -> Gain80/1
  Power (Phasor)35/2 -> Gain76/1
  Demux22/1 -> Power (Phasor)35/1
  Power (Phasor)34/1 -> Gain79/1
  [I830] -> To Workspace27/1, Demux23/1
  [I854] -> To Workspace29/1, Demux25/1
  Demux25/2 -> Power (Phasor)36/2
  Power (Phasor)38/1 -> Gain81/1
  [V854] -> To Workspace28/1, Demux24/1
  Power (Phasor)37/1 -> Gain85/1
  Power (Phasor)37/2 -> Gain86/1
  Gain81/1 -> Display81/1
  Gain86/1 -> Display86/1
  Gain85/1 -> Display85/1
  Gain83/1 -> Display83/1
  Demux24/3 -> Power (Phasor)37/1
  Demux24/1 -> Power (Phasor)38/1
  Gain82/1 -> Display82/1
  Power (Phasor)36/1 -> Gain83/1
  Demux25/3 -> Power (Phasor)37/2
  Power (Phasor)36/2 -> Gain84/1
  Power (Phasor)38/2 -> Gain82/1
  Demux25/1 -> Power (Phasor)38/2
  Demux24/2 -> Power (Phasor)36/1
  Gain84/1 -> Display84/1
  Gain90/1 -> Display90/1
  Power (Phasor)39/1 -> Gain89/1
  Power (Phasor)41/2 -> Gain88/1
  Demux27/1 -> Power (Phasor)41/2
  Demux27/3 -> Power (Phasor)40/2
  Demux26/2 -> Power (Phasor)39/1
  Power (Phasor)39/2 -> Gain90/1
  [I852] -> To Workspace31/1, Demux27/1
  Gain91/1 -> Display91/1
  Gain88/1 -> Display88/1
  Demux26/3 -> Power (Phasor)40/1
  Gain89/1 -> Display89/1
  Gain92/1 -> Display92/1
  Power (Phasor)41/1 -> Gain87/1
  [V852] -> To Workspace30/1, Demux26/1
  Demux27/2 -> Power (Phasor)39/2
  Power (Phasor)40/2 -> Gain92/1
  Power (Phasor)40/1 -> Gain91/1
  Demux26/1 -> Power (Phasor)41/1
  Gain87/1 -> Display87/1
  Gain98/1 -> Display98/1
  Gain94/1 -> Display94/1
  Gain95/1 -> Display95/1
  Demux28/3 -> Power (Phasor)43/1
  Gain97/1 -> Display97/1
  [IRG11] -> To Workspace33/1, Demux29/1
  Power (Phasor)42/2 -> Gain96/1
  Demux29/3 -> Power (Phasor)43/2
  Demux29/1 -> Power (Phasor)44/2
  Power (Phasor)42/1 -> Gain95/1
  Power (Phasor)44/2 -> Gain94/1
  Gain96/1 -> Display96/1
  Demux28/1 -> Power (Phasor)44/1
  Demux28/2 -> Power (Phasor)42/1
  Power (Phasor)43/2 -> Gain98/1
  Power (Phasor)43/1 -> Gain97/1
  Gain93/1 -> Display93/1
  Demux29/2 -> Power (Phasor)42/2
  Power (Phasor)44/1 -> Gain93/1
  [VRG11] -> To Workspace32/1, Demux28/1
  Demux32/1 -> Power (Phasor)50/1
  Gain105/1 -> Display105/1
  Power (Phasor)50/2 -> Gain106/1
  [I818] -> To Workspace17/1, Demux33/1
  Power (Phasor)50/1 -> Gain105/1
  Gain106/1 -> Display106/1
  Power (Phasor)49/2 -> Gain110/1
  Gain110/1 -> Display110/1
  [V818] -> To Workspace16/1, Demux32/1
  Gain109/1 -> Display109/1
  Gain107/1 -> Display107/1
  Demux33/2 -> Power (Phasor)48/2
  Demux32/2 -> Power (Phasor)48/1
  Demux32/3 -> Power (Phasor)49/1
  Power (Phasor)48/2 -> Gain108/1
  Demux33/1 -> Power (Phasor)50/2
  Power (Phasor)49/1 -> Gain109/1
  Demux33/3 -> Power (Phasor)49/2
  Power (Phasor)48/1 -> Gain107/1
  Gain108/1 -> Display108/1
  Demux34/1 -> Power (Phasor)53/1
  Gain111/1 -> Display111/1
  Power (Phasor)53/2 -> Gain112/1
  [I820] -> To Workspace19/1, Demux35/1
  Power (Phasor)53/1 -> Gain111/1
  Gain112/1 -> Display112/1
  Power (Phasor)52/2 -> Gain116/1
  Gain116/1 -> Display116/1
  [V820] -> To Workspace18/1, Demux34/1
  Gain115/1 -> Display115/1
  Gain113/1 -> Display113/1
  Demux35/2 -> Power (Phasor)51/2
  Demux34/2 -> Power (Phasor)51/1
  Demux34/3 -> Power (Phasor)52/1
  Power (Phasor)51/2 -> Gain114/1
  Demux35/1 -> Power (Phasor)53/2
  Power (Phasor)52/1 -> Gain115/1
  Demux35/3 -> Power (Phasor)52/2
  Power (Phasor)51/1 -> Gain113/1
  Gain114/1 -> Display114/1
  Gain120/1 -> Display120/1
  Demux37/3 -> Power (Phasor)55/2
  Power (Phasor)54/1 -> Gain119/1
  Power (Phasor)54/2 -> Gain120/1
  Power (Phasor)55/1 -> Gain121/1
  Demux36/3 -> Power (Phasor)55/1
  Gain119/1 -> Display119/1
  Demux37/1 -> Power (Phasor)56/2
  Demux36/2 -> Power (Phasor)54/1
  Demux37/2 -> Power (Phasor)54/2
  [V822] -> To Workspace20/1, Demux36/1
  Gain117/1 -> Display117/1
  Power (Phasor)56/2 -> Gain118/1
  Demux36/1 -> Power (Phasor)56/1
  Power (Phasor)56/1 -> Gain117/1
  Gain122/1 -> Display122/1
  Gain118/1 -> Display118/1
  Power (Phasor)55/2 -> Gain122/1
  [I822] -> To Workspace21/1, Demux37/1
  Gain121/1 -> Display121/1
  Demux31/2 -> Power (Phasor)45/2
  [I832] -> To Workspace35/1, Demux31/1
  Demux31/3 -> Power (Phasor)46/2
  Gain137/1 -> Display137/1
  Gain101/1 -> Display101/1
  [V832] -> To Workspace34/1, Demux30/1
  Demux30/2 -> Power (Phasor)45/1
  Demux30/3 -> Power (Phasor)46/1
  Gain103/1 -> Display103/1
  Power (Phasor)47/1 -> Gain137/1
  Power (Phasor)45/1 -> Gain101/1
  Power (Phasor)46/2 -> Gain104/1
  Power (Phasor)45/2 -> Gain102/1
  Power (Phasor)46/1 -> Gain103/1
  Gain102/1 -> Display102/1
  Demux30/1 -> Power (Phasor)47/1
  Power (Phasor)47/2 -> Gain100/1
  Gain104/1 -> Display104/1
  Demux31/1 -> Power (Phasor)47/2
  Gain100/1 -> Display100/1

== system T2F_IEEE34bus_v2019b_Phasor_PI_ZIPload/Regulator 1/Single Phase SVR_A ==
  Line Drop Compensator : Subsystem
  Transformer with Taps : Subsystem
  Voltage Regulator Control : Subsystem
  S : PMIOPort  Tag=PMCPort  Side=Left
  L : PMIOPort  Tag=PMCPort  Port=2  Side=Right
  Tap : Outport  VectorParamsAs1DForOutWhenUnconnected=off
  tag scope: Vr1a=global
  wires:
  Line Drop Compensator/1(Vm) -> [Vr1a], Voltage Regulator Control/1(Vm)
  Voltage Regulator Control/1(Tap) -> Transformer with Taps/1(tap), Tap/1
  Transformer with Taps/1(Isec) -> Line Drop Compensator/1(Isec)
  Transformer with Taps/2(Vsec) -> Line Drop Compensator/2(Vsec)
  connections:
  Transformer with Taps/RConn1 -- L/RConn1
  Transformer with Taps/LConn1 -- S/RConn1

== system T2F_IEEE34bus_v2019b_Phasor_PI_ZIPload/Regulator 1/Single Phase SVR_B ==
  Line Drop Compensator : Subsystem
  Transformer with Taps : Subsystem
  Voltage Regulator Control : Subsystem
  S : PMIOPort  Tag=PMCPort  Side=Left
  L : PMIOPort  Tag=PMCPort  Port=2  Side=Right
  Tap : Outport  VectorParamsAs1DForOutWhenUnconnected=off
  tag scope: Vr1b=global
  wires:
  Transformer with Taps/2(Vsec) -> Line Drop Compensator/2(Vsec)
  Transformer with Taps/1(Isec) -> Line Drop Compensator/1(Isec)
  Voltage Regulator Control/1(Tap) -> Transformer with Taps/1(tap), Tap/1
  Line Drop Compensator/1(Vm) -> [Vr1b], Voltage Regulator Control/1(Vm)
  connections:
  Transformer with Taps/LConn1 -- S/RConn1
  Transformer with Taps/RConn1 -- L/RConn1

== system T2F_IEEE34bus_v2019b_Phasor_PI_ZIPload/Regulator 1/Single Phase SVR_C ==
  Line Drop Compensator : Subsystem
  Transformer with Taps : Subsystem
  Voltage Regulator Control : Subsystem
  S : PMIOPort  Tag=PMCPort  Side=Left
  L : PMIOPort  Tag=PMCPort  Port=2  Side=Right
  Tap : Outport  VectorParamsAs1DForOutWhenUnconnected=off
  tag scope: Vr1c=global
  wires:
  Line Drop Compensator/1(Vm) -> [Vr1c], Voltage Regulator Control/1(Vm)
  Voltage Regulator Control/1(Tap) -> Transformer with Taps/1(tap), Tap/1
  Transformer with Taps/1(Isec) -> Line Drop Compensator/1(Isec)
  Transformer with Taps/2(Vsec) -> Line Drop Compensator/2(Vsec)
  connections:
  Transformer with Taps/RConn1 -- L/RConn1
  Transformer with Taps/LConn1 -- S/RConn1

== system T2F_IEEE34bus_v2019b_Phasor_PI_ZIPload/Regulator 2/Single Phase SVR_A ==
  Line Drop Compensator : Subsystem
  Transformer with Taps : Subsystem
  Voltage Regulator Control : Subsystem
  S : PMIOPort  Tag=PMCPort  Side=Left
  L : PMIOPort  Tag=PMCPort  Port=2  Side=Right
  Tap : Outport  VectorParamsAs1DForOutWhenUnconnected=off
  tag scope: Vr2a=global
  wires:
  Line Drop Compensator/1(Vm) -> [Vr2a], Voltage Regulator Control/1(Vm)
  Voltage Regulator Control/1(Tap) -> Transformer with Taps/1(tap), Tap/1
  Transformer with Taps/1(Isec) -> Line Drop Compensator/1(Isec)
  Transformer with Taps/2(Vsec) -> Line Drop Compensator/2(Vsec)
  connections:
  Transformer with Taps/RConn1 -- L/RConn1
  Transformer with Taps/LConn1 -- S/RConn1

== system T2F_IEEE34bus_v2019b_Phasor_PI_ZIPload/Regulator 2/Single Phase SVR_B ==
  Line Drop Compensator : Subsystem
  Transformer with Taps : Subsystem
  Voltage Regulator Control : Subsystem
  S : PMIOPort  Tag=PMCPort  Side=Left
  L : PMIOPort  Tag=PMCPort  Port=2  Side=Right
  Tap : Outport  VectorParamsAs1DForOutWhenUnconnected=off
  tag scope: Vr2b=global
  wires:
  Transformer with Taps/2(Vsec) -> Line Drop Compensator/2(Vsec)
  Transformer with Taps/1(Isec) -> Line Drop Compensator/1(Isec)
  Voltage Regulator Control/1(Tap) -> Transformer with Taps/1(tap), Tap/1
  Line Drop Compensator/1(Vm) -> [Vr2b], Voltage Regulator Control/1(Vm)
  connections:
  Transformer with Taps/LConn1 -- S/RConn1
  Transformer with Taps/RConn1 -- L/RConn1

== system T2F_IEEE34bus_v2019b_Phasor_PI_ZIPload/Regulator 2/Single Phase SVR_C ==
  Line Drop Compensator : Subsystem
  Transformer with Taps : Subsystem
  Voltage Regulator Control : Subsystem
  S : PMIOPort  Tag=PMCPort  Side=Left
  L : PMIOPort  Tag=PMCPort  Port=2  Side=Right
  Tap : Outport  VectorParamsAs1DForOutWhenUnconnected=off
  tag scope: Vr2c=global
  wires:
  Line Drop Compensator/1(Vm) -> [Vr2c], Voltage Regulator Control/1(Vm)
  Voltage Regulator Control/1(Tap) -> Transformer with Taps/1(tap), Tap/1
  Transformer with Taps/1(Isec) -> Line Drop Compensator/1(Isec)
  Transformer with Taps/2(Vsec) -> Line Drop Compensator/2(Vsec)
  connections:
  Transformer with Taps/RConn1 -- L/RConn1
  Transformer with Taps/LConn1 -- S/RConn1

== system T2F_IEEE34bus_v2019b_Phasor_PI_ZIPload/Regulator 1/Single Phase SVR_A/Line Drop Compensator ==
  note: Vm=Vsec-Isec(Rc+jXc)
  Isec : Inport
  Vsec : Inport  Port=2
  Abs1 : Abs  SaturateOnIntegerOverflow=off
  Gain4 : Gain  Gain=1/sqrt(2)
  Gain5 : Gain  Gain=Rc+j*Xc
  Gain6 : Gain  Gain=1/sqrt(2)
  Sum1 : Sum  Inputs=|+-
  Vm : Outport
  wires:
  Abs1/1 -> Vm/1
  Sum1/1 -> Abs1/1
  Isec/1 -> Gain4/1
  Vsec/1 -> Gain6/1
  Gain4/1 -> Gain5/1
  Gain6/1 -> Sum1/1
  Gain5/1 -> Sum1/2
